simulink model "UltrasoundPipelineDiagram"  (R2024b)
settings: Solver=VariableStepAuto  StartTime=0.0  StopTime=10.0  RelTol=1e-3
settings Model: Creator=rohit  LastModifiedBy=rohit

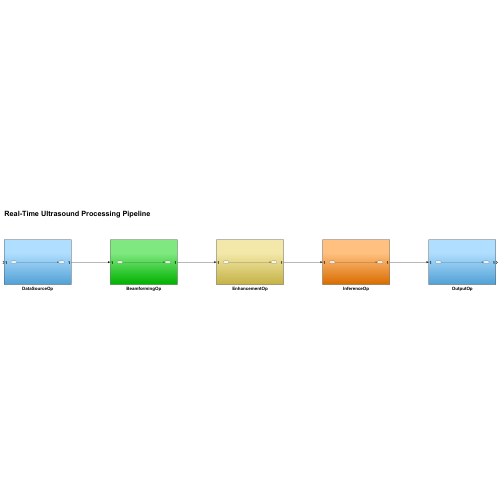
[thumbnail: Simulink's stored preview of the top-level diagram]
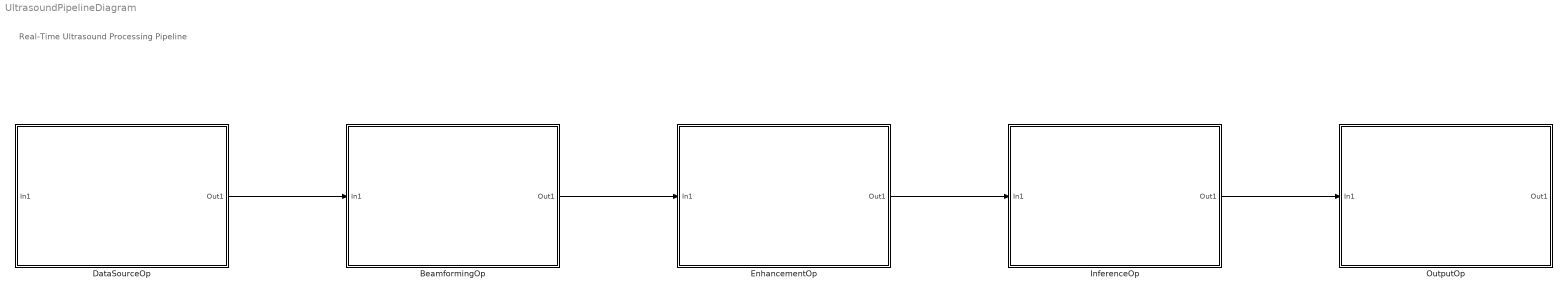
== system UltrasoundPipelineDiagram ==
  note: Real-Time Ultrasound Processing Pipeline
  BeamformingOp : Subsystem
  DataSourceOp : Subsystem
  EnhancementOp : Subsystem
  InferenceOp : Subsystem
  OutputOp : Subsystem
  wires:
  DataSourceOp/1(Out1) -> BeamformingOp/1(In1)
  BeamformingOp/1(Out1) -> EnhancementOp/1(In1)
  EnhancementOp/1(Out1) -> InferenceOp/1(In1)
  InferenceOp/1(Out1) -> OutputOp/1(In1)

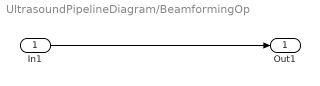
== system UltrasoundPipelineDiagram/BeamformingOp ==
  In1 : Inport
  Out1 : Outport
  wires:
  In1/1 -> Out1/1

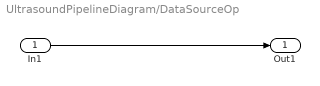
== system UltrasoundPipelineDiagram/DataSourceOp ==
  In1 : Inport
  Out1 : Outport
  wires:
  In1/1 -> Out1/1

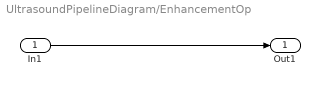
== system UltrasoundPipelineDiagram/EnhancementOp ==
  In1 : Inport
  Out1 : Outport
  wires:
  In1/1 -> Out1/1

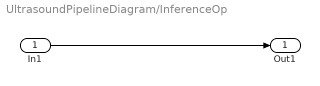
== system UltrasoundPipelineDiagram/InferenceOp ==
  In1 : Inport
  Out1 : Outport
  wires:
  In1/1 -> Out1/1

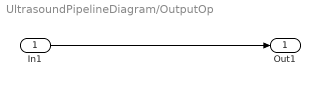
== system UltrasoundPipelineDiagram/OutputOp ==
  In1 : Inport
  Out1 : Outport
  wires:
  In1/1 -> Out1/1
